simulink model "close_loop_rollpitchyaw"  (R2018b)
settings: Solver=VariableStepAuto  StartTime=0.0  StopTime=5  RelTol=1e-3
libraries: simulink x3
settings Model: Creator=ewert  LastModifiedBy=cnit355
settings SFSimCC: SimUseLocalCustomCode=off
settings RTWCC: RTWUseLocalCustomCode=off
settings CodeAppCC: StateflowObjectComments=on

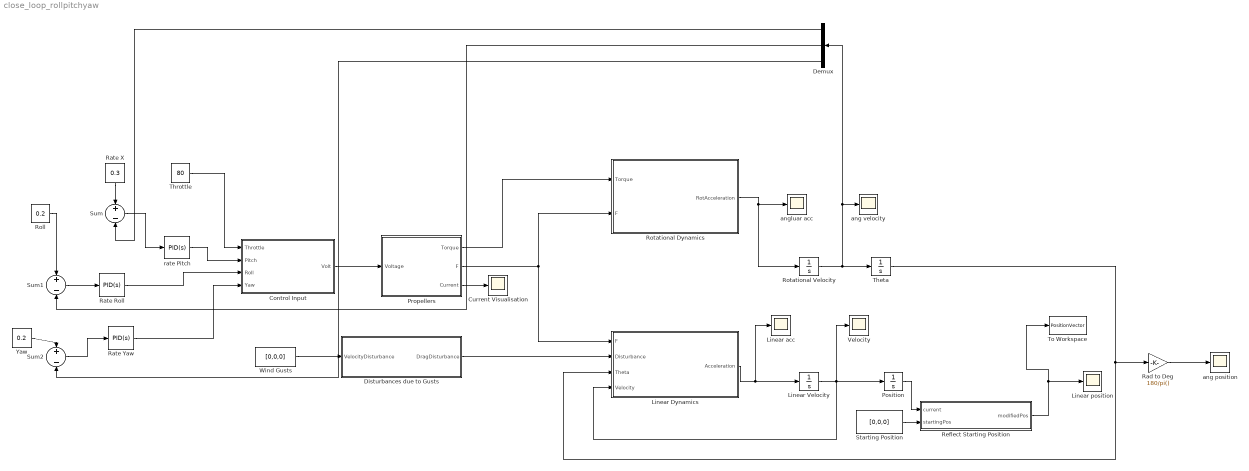
== system close_loop_rollpitchyaw ==
  " Control Input" : MATLAB Function  TreatAsAtomicUnit=on
  "Current Visualisation " : Scope
  Demux : Demux  Outputs=3
  Disturbances due to Gusts : MATLAB Function  TreatAsAtomicUnit=on
  Linear Dynamics : MATLAB Function  TreatAsAtomicUnit=on
  Linear Velocity : Integrator
  Linear acc : Scope
  Linear position : Scope
  Position : Integrator
  Propellers : MATLAB Function  TreatAsAtomicUnit=on
  Rad to Deg : Gain  Gain=180/pi()
  Rate Roll : simulink/Continuous/PID Controller  Controller=PID  Form=Parallel  TimeDomain=Continuous-time  SampleTime=-1  IntegratorMethod=Forward Euler  FilterMethod=Forward Euler  ControllerParametersSource=internal  P=10  I=5  D=0  UseFilter=on  N=100  TunerSelectOption=Transfer Function Based (PID Tuner App)  InitialConditionSource=internal  InitialConditionForIntegrator=0  InitialConditionForFilter=0  DifferentiatorICPrevScaledInput=0  ExternalReset=none  TrackingMode=off  Kt=1  LimitOutput=on  UpperSaturationLimit=100  LowerSaturationLimit=0  LinearizeAsGain=on  AntiWindupMode=clamping  Kb=1  POutMin=[]  POutMax=[]  IOutMin=[]  IOutMax=[]  DOutMin=[]  DOutMax=[]  NOutMin=[]  NOutMax=[]  SumOutMin=[]  SumOutMax=[]  SaturationOutMin=[]  SaturationOutMax=[]  PParamMin=[]  PParamMax=[]  IParamMin=[]  IParamMax=[]  DParamMin=[]  DParamMax=[]  NParamMin=[]  NParamMax=[]  KbParamMin=[]  KbParamMax=[]  KtParamMin=[]  KtParamMax=[]  KbOutMin=[]  KbOutMax=[]  KtOutMin=[]  KtOutMax=[]  IntegratorOutMin=[]  IntegratorOutMax=[]  FilterOutMin=[]  FilterOutMax=[]  SumI1OutMin=[]  SumI1OutMax=[]  SumI2OutMin=[]  SumI2OutMax=[]  SumI3OutMin=[]  SumI3OutMax=[]  SumI4OutMin=[]  SumI4OutMax=[]  SumDOutMin=[]  SumDOutMax=[]  DifferentiatorOutMin=[]  DifferentiatorOutMax=[]  FilterDiffOutCoefMin=[]  FilterDiffOutCoefMax=[]  ReciprocalOutMin=[]  ReciprocalOutMax=[]  SumDenOutMin=[]  SumDenOutMax=[]  SumNumOutMin=[]  SumNumOutMax=[]  DivideOutMin=[]  DivideOutMax=[]  IntegratorContinuousStateAttributes=''  IntegratorStateMustResolveToSignalObject=off  IntegratorRTWStateStorageClass=Auto  FilterContinuousStateAttributes=''  FilterStateMustResolveToSignalObject=off  FilterRTWStateStorageClass=Auto  ParallelPVariant=InternalParameters  IdealPVariant=Disabled  IVariant=InternalParameters  DVariant=InternalParameters  IntegratorVariant=Continuous  SatVariant=Enabled  AWVariant=ContClampingParallel  PCopyVariant=Disabled  TRVariant=Disabled  FdbkBlocksVariant=Forward  IdealPFdbkVariant=Disabled  SatFdbkVariant=Disabled  DerivativeFilterVariant=ContFilter  NVariant=InternalParameters  NCopyVariant=Disabled  FilterICVariant=InternalICsFilter  IntegratorICVariant=InternalICs  ExternalResetVariant=Disabled  TRSumVariant=Passthrough  SumFdbkVariant=Disabled  SumVariant=Sum_PID
  Rate X : Constant  Value=0.3
  Rate Yaw : simulink/Continuous/PID Controller  Controller=PID  Form=Parallel  TimeDomain=Continuous-time  SampleTime=-1  IntegratorMethod=Forward Euler  FilterMethod=Forward Euler  ControllerParametersSource=internal  P=5  I=0.5  D=0  UseFilter=on  N=100  TunerSelectOption=Transfer Function Based (PID Tuner App)  InitialConditionSource=internal  InitialConditionForIntegrator=0  InitialConditionForFilter=0  DifferentiatorICPrevScaledInput=0  ExternalReset=none  TrackingMode=off  Kt=1  LimitOutput=on  UpperSaturationLimit=100  LowerSaturationLimit=0  LinearizeAsGain=on  AntiWindupMode=clamping  Kb=1  POutMin=[]  POutMax=[]  IOutMin=[]  IOutMax=[]  DOutMin=[]  DOutMax=[]  NOutMin=[]  NOutMax=[]  SumOutMin=[]  SumOutMax=[]  SaturationOutMin=[]  SaturationOutMax=[]  PParamMin=[]  PParamMax=[]  IParamMin=[]  IParamMax=[]  DParamMin=[]  DParamMax=[]  NParamMin=[]  NParamMax=[]  KbParamMin=[]  KbParamMax=[]  KtParamMin=[]  KtParamMax=[]  KbOutMin=[]  KbOutMax=[]  KtOutMin=[]  KtOutMax=[]  IntegratorOutMin=[]  IntegratorOutMax=[]  FilterOutMin=[]  FilterOutMax=[]  SumI1OutMin=[]  SumI1OutMax=[]  SumI2OutMin=[]  SumI2OutMax=[]  SumI3OutMin=[]  SumI3OutMax=[]  SumI4OutMin=[]  SumI4OutMax=[]  SumDOutMin=[]  SumDOutMax=[]  DifferentiatorOutMin=[]  DifferentiatorOutMax=[]  FilterDiffOutCoefMin=[]  FilterDiffOutCoefMax=[]  ReciprocalOutMin=[]  ReciprocalOutMax=[]  SumDenOutMin=[]  SumDenOutMax=[]  SumNumOutMin=[]  SumNumOutMax=[]  DivideOutMin=[]  DivideOutMax=[]  IntegratorContinuousStateAttributes=''  IntegratorStateMustResolveToSignalObject=off  IntegratorRTWStateStorageClass=Auto  FilterContinuousStateAttributes=''  FilterStateMustResolveToSignalObject=off  FilterRTWStateStorageClass=Auto  ParallelPVariant=InternalParameters  IdealPVariant=Disabled  IVariant=InternalParameters  DVariant=InternalParameters  IntegratorVariant=Continuous  SatVariant=Enabled  AWVariant=ContClampingParallel  PCopyVariant=Disabled  TRVariant=Disabled  FdbkBlocksVariant=Forward  IdealPFdbkVariant=Disabled  SatFdbkVariant=Disabled  DerivativeFilterVariant=ContFilter  NVariant=InternalParameters  NCopyVariant=Disabled  FilterICVariant=InternalICsFilter  IntegratorICVariant=InternalICs  ExternalResetVariant=Disabled  TRSumVariant=Passthrough  SumFdbkVariant=Disabled  SumVariant=Sum_PID
  Reflect Starting Position : MATLAB Function  TreatAsAtomicUnit=on
  Roll : Constant  Value=0.2
  Rotational Dynamics : MATLAB Function  TreatAsAtomicUnit=on
  Rotational Velocity : Integrator
  Starting Position : Constant  Value=[0,0,0]  VectorParams1D=off
  Sum : Sum  Inputs=+-
  Sum1 : Sum  Inputs=+-
  Sum2 : Sum  Inputs=+-
  Theta : Integrator
  Throttle : Constant  Value=80
  To Workspace : ToWorkspace  VariableName=PositionVector  SampleTime=-1
      settings: Save2DSignal=2-D array (concatenate along first dimension)
  "Velocity " : Scope
  Wind Gusts : Constant  Value=[0,0,0]
  Yaw : Constant  Value=0.2
  ang position : Scope
  ang velocity : Scope
  angluar acc : Scope
  rate Pitch : simulink/Continuous/PID Controller  Controller=PID  Form=Parallel  TimeDomain=Continuous-time  SampleTime=-1  IntegratorMethod=Forward Euler  FilterMethod=Forward Euler  ControllerParametersSource=internal  P=10  I=5  D=0  UseFilter=on  N=100  TunerSelectOption=Transfer Function Based (PID Tuner App)  InitialConditionSource=internal  InitialConditionForIntegrator=0  InitialConditionForFilter=0  DifferentiatorICPrevScaledInput=0  ExternalReset=none  TrackingMode=off  Kt=1  LimitOutput=on  UpperSaturationLimit=100  LowerSaturationLimit=0  LinearizeAsGain=on  AntiWindupMode=clamping  Kb=1  POutMin=[]  POutMax=[]  IOutMin=[]  IOutMax=[]  DOutMin=[]  DOutMax=[]  NOutMin=[]  NOutMax=[]  SumOutMin=[]  SumOutMax=[]  SaturationOutMin=[]  SaturationOutMax=[]  PParamMin=[]  PParamMax=[]  IParamMin=[]  IParamMax=[]  DParamMin=[]  DParamMax=[]  NParamMin=[]  NParamMax=[]  KbParamMin=[]  KbParamMax=[]  KtParamMin=[]  KtParamMax=[]  KbOutMin=[]  KbOutMax=[]  KtOutMin=[]  KtOutMax=[]  IntegratorOutMin=[]  IntegratorOutMax=[]  FilterOutMin=[]  FilterOutMax=[]  SumI1OutMin=[]  SumI1OutMax=[]  SumI2OutMin=[]  SumI2OutMax=[]  SumI3OutMin=[]  SumI3OutMax=[]  SumI4OutMin=[]  SumI4OutMax=[]  SumDOutMin=[]  SumDOutMax=[]  DifferentiatorOutMin=[]  DifferentiatorOutMax=[]  FilterDiffOutCoefMin=[]  FilterDiffOutCoefMax=[]  ReciprocalOutMin=[]  ReciprocalOutMax=[]  SumDenOutMin=[]  SumDenOutMax=[]  SumNumOutMin=[]  SumNumOutMax=[]  DivideOutMin=[]  DivideOutMax=[]  IntegratorContinuousStateAttributes=''  IntegratorStateMustResolveToSignalObject=off  IntegratorRTWStateStorageClass=Auto  FilterContinuousStateAttributes=''  FilterStateMustResolveToSignalObject=off  FilterRTWStateStorageClass=Auto  ParallelPVariant=InternalParameters  IdealPVariant=Disabled  IVariant=InternalParameters  DVariant=InternalParameters  IntegratorVariant=Continuous  SatVariant=Enabled  AWVariant=ContClampingParallel  PCopyVariant=Disabled  TRVariant=Disabled  FdbkBlocksVariant=Forward  IdealPFdbkVariant=Disabled  SatFdbkVariant=Disabled  DerivativeFilterVariant=ContFilter  NVariant=InternalParameters  NCopyVariant=Disabled  FilterICVariant=InternalICsFilter  IntegratorICVariant=InternalICs  ExternalResetVariant=Disabled  TRSumVariant=Passthrough  SumFdbkVariant=Disabled  SumVariant=Sum_PID
  wires:
  Propellers/1(Torque) -> Rotational Dynamics/1(Torque)
  Propellers/2(F) -> Linear Dynamics/1(F), Rotational Dynamics/2(F)
  Rotational Dynamics/1(RotAcceleration) -> Rotational Velocity/1, angluar acc/1
  Rotational Velocity/1 -> Demux/1, ang velocity/1, Theta/1
  Theta/1 -> Linear Dynamics/3(Theta), Rad to Deg/1
  Linear Dynamics/1(Acceleration) -> Linear acc/1, Linear Velocity/1
  Linear Velocity/1 -> "Velocity "/1, Position/1, Linear Dynamics/4(Velocity)
  Disturbances due to Gusts/1(DragDisturbance) -> Linear Dynamics/2(Disturbance)
  Wind Gusts/1 -> Disturbances due to Gusts/1(VelocityDisturbance)
  " Control Input"/1(Volt) -> Propellers/1(Voltage)
  Rad to Deg/1 -> ang position/1
  Propellers/3(Current) -> "Current Visualisation "/1
  Rate X/1 -> Sum/1
  Sum/1 -> rate Pitch/1
  Demux/1 -> Sum/2
  Throttle/1 -> " Control Input"/1(Throttle)
  Roll/1 -> Sum1/1
  Sum1/1 -> Rate Roll/1
  Demux/2 -> Sum1/2
  Yaw/1 -> Sum2/1
  Sum2/1 -> Rate Yaw/1
  Demux/3 -> Sum2/2
  rate Pitch/1 -> " Control Input"/2(Pitch)
  Rate Roll/1 -> " Control Input"/3(Roll)
  Rate Yaw/1 -> " Control Input"/4(Yaw)
  Position/1 -> Reflect Starting Position/1(current)
  Starting Position/1 -> Reflect Starting Position/2(startingPos)
  Reflect Starting Position/1(modifiedPos) -> To Workspace/1, Linear position/1

== matlab function close_loop_rollpitchyaw/Rotational Dynamics ==
  data: Torque input; RotAcceleration output; F input
function RotAcceleration = fcn(Torque, F)
Moment = [0 0 0];
RotAcceleration = [0 0 0]; 
Inertia = [0.003, 0.003, 0.007]; %moment of inertia

Moment(1) =  (F(3)+F(4)) * 0.237/2 - (F(1)+F(2))*0.237/2;
Moment(2) =  (F(3)+F(2)) * 0.237/2 - (F(1)+F(4))*0.237/2;
Moment(3) =  Torque(4) - Torque(1) + Torque(2) - Torque(3); %yaw

for i=1:3
    RotAcceleration(i) = Moment(i) / Inertia(i);
end

== matlab function close_loop_rollpitchyaw/Propellers ==
  data: Voltage input; Torque output; F output; Current output
function [Torque, F, Current] = fcn(Voltage)

RPM = [0 0 0 0];
Torque = [0 0 0 0];
Current = [0 0 0 0];
F = [0 0 0 0];

for i=1:4
    RPM(i) = -2.6931*Voltage(i)^3 + 1400*Voltage(i);
    Ct = 2 * (10^-15) * (RPM(i)^3) - 4 * (10^-11) * (RPM(i)^2) + 3 * (10^(-7)) * RPM(i) + 0.1013;
    F(i) = Ct * 1.225*(RPM(i)/60)^2 * 0.2^4; %0.2 = diameter of propeller
    Torque(i) = 4 * 10^-14 * RPM(i)^3 + 8 * 10^-12 * RPM(i)^2 + 3 * 10^-6 * RPM(i);
    Current(i) = 1400*Torque(i);
end

== matlab function close_loop_rollpitchyaw/Linear Dynamics ==
  data: F input; Acceleration output; Disturbance input; Theta input; Velocity input
function Acceleration  = fcn(F,Disturbance,Theta,Velocity)
m=0.743; %mass
g=9.81; %gravity
A=[0.0197 0.0197 0.0512]; %projected area 
air=1.225; %air density
Cd=1; %coefficient of drag

Acceleration=[0 0 0];
Force = [0 0 0];
Fprop = [0 0 0]; %thrust in x,y,z direction
% Prop=[0;0;0];

Fprop(1)=sin(Theta(2))*cos(Theta(1))*(F(1)+F(2)+F(3)+F(4));
Fprop(2)=sin(Theta(1))*cos(Theta(2))*(F(1)+F(2)+F(3)+F(4));
Fprop(3)=cos(Theta(1))*cos(Theta(2))*(F(1)+F(2)+F(3)+F(4));
% Prop(1,1)=sin(Theta(2))*cos(Theta(1))*(F(1)+F(2)+F(3)+F(4));
% Prop(2,1)=sin(Theta(1))*cos(Theta(2))*(F(1)+F(2)+F(3)+F(4));
% Prop(3,1)=(F(1)+F(2)+F(3)+F(4))*cos(Theta(1))*cos(Theta(2));

ThetaXY = -atan2(Fprop(1),Fprop(2));
XY2D=sqrt(Fprop(1)^2+Fprop(2)^2); %thrust projection vector

%Yaw 
if Fprop(3)>=0
    Fprop(1)=XY2D*sin(Theta(3)+ThetaXY); %magnitude of 2d vector * sign(angle + yaw motion)
    Fprop(2)=XY2D*cos(Theta(3)+ThetaXY);
else
     Fprop(1)=XY2D*sin(-Theta(3)+ThetaXY);
    Fprop(2)=XY2D*cos(-Theta(3)+ThetaXY);
end

%+ - drag based on move forward/ backward
if Velocity(1)<0
    Force(1)=Fprop(1)-Disturbance(1)+0.5*air*Velocity(1)^2*A(1)*Cd;
else 
    Force(1)=Fprop(1)-Disturbance(1)-0.5*air*Velocity(1)^2*A(1)*Cd;
end

if Velocity(2)<0
    Force(2)=Fprop(2)-Disturbance(2)+0.5*air*Velocity(2)^2*A(2)*Cd;
else 
    Force(2)=Fprop(2)-Disturbance(2)-0.5*air*Velocity(2)^2*A(2)*Cd;
end

if Velocity(3)<0
    Force(3)=Fprop(3)+0.5*air*Velocity(3)^2*A(3)*Cd-m*g-Disturbance(3);
else 
    Force(3)=Fprop(3)-0.5*air*Velocity(3)^2*A(3)*Cd-m*g-Disturbance(3);
end

disp("FORCE")
disp(Force)
for i=1:3
    Acceleration(i)=Force(i)/m;
end

== matlab function close_loop_rollpitchyaw/Disturbances due to Gusts ==
  data: VelocityDisturbance input; DragDisturbance output
function DragDisturbance = fcn(VelocityDisturbance)
A=[0.0197 0.0197 0.0197*2*1.3];
DragDisturbance=[0 0 0];
rho=1.225;
Cd=1;

for i=1:3
    if VelocityDisturbance(i)<0
        DragDisturbance(i)=-0.5*rho*VelocityDisturbance(i)^2*A(i)*Cd;
    else
        DragDisturbance(i)=0.5*rho*VelocityDisturbance(i)^2*A(i)*Cd;
    end
end

== matlab function close_loop_rollpitchyaw/ Control Input ==
  data: Throttle input; Volt output; Pitch input; Roll input; Yaw input
function Volt = fcn(Throttle, Pitch, Roll, Yaw)

Correct = 0; %correction of final voltage
%increase, decrease throttle level that symmetry works

%condition of each input 
%Throttle <- increase and decrease pitch roll yaw symetrically
if (Pitch/2+Roll/2+Yaw/2) > (100-Throttle) % -50 ~ +50
   
    Correct = ((Pitch/2 + Roll/2 + Yaw/2) - (100 - Throttle));
       
end

if Throttle > 10 && (Pitch/2+Roll/2+Yaw/2) > (Throttle-10) %Enough space for other size // make it never go down to 10%... -10 will result in false movement

    if Correct < ((Pitch/2 + Roll/2 + Yaw/2) - (Throttle - 10)) % jf too big, take excess
        Correct = ((Pitch/2 + Roll/2 + Yaw/2) - (Throttle - 10)) ;   
    end
            
end

if Correct ~= 0 
    %Correct pitch, roll, yaw from user input
    Pitch = Pitch - Correct / 3 * 2; %distribute excess to pitch, roll, and yaw
    Roll = Roll - Correct / 3 * 2;
    Yaw = Yaw - Correct / 3 * 2;
end

%voltage for each motor
Volt = [(Throttle - Pitch / 2 - Roll / 2 - Yaw / 2)*11.4/100 %percent=> divide by 100 /  voltage max = 11.4
    (Throttle - Pitch / 2 + Roll / 2 + Yaw / 2)*11.4/100
    (Throttle + Pitch / 2 + Roll / 2 - Yaw / 2)*11.4/100
    (Throttle + Pitch / 2 - Roll / 2 + Yaw / 2)*11.4/100];

== matlab function close_loop_rollpitchyaw/Reflect Starting Position ==
  data: current input; modifiedPos output; startingPos input
function modifiedPos = fcn(current, startingPos)
modifiedPos = current + startingPos;
